simulink model "shifter_system_sim"  (R2018a)
settings: Solver=VariableStepAuto  StartTime=0.0  StopTime=3  RelTol=1e-3
libraries: simulink x2, dspstat3 x1
settings Model: Creator=m_tam  LastModifiedBy=m_tam

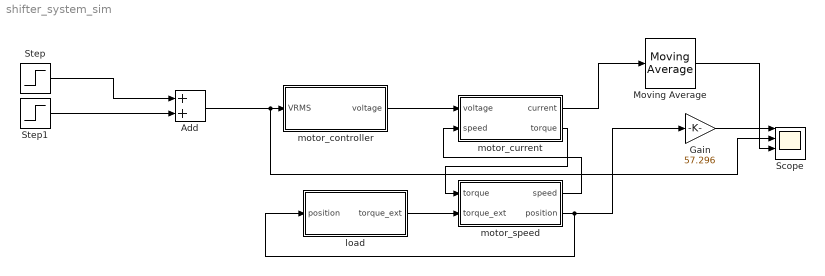
== system shifter_system_sim ==
  Add : Sum
  Gain : Gain  Gain=57.296
  Moving Average : dspstat3/Moving Average  Method=Exponential weighting  ForgettingFactorPort=off  SpecifyWindowLength=on  WindowLength=1000  ForgettingFactor=.999  SimulateUsing=Code generation
  Scope : Scope  NumInputPorts=4
  Step : Step  After=1.125  SampleTime=0
  Step1 : Step  Time=2  After=3  SampleTime=0
  load : Subsystem
  motor_controller : Subsystem
  motor_current : Subsystem
  motor_speed : Subsystem
  wires:
  motor_speed/1(speed) -> motor_current/2(speed)
  motor_speed/2(position) -> load/1(position), Gain/1
  motor_current/2(torque) -> motor_speed/1(torque)
  load/1(torque_ext) -> motor_speed/2(torque_ext)
  motor_controller/1(voltage) -> motor_current/1(voltage)
  Add/1 -> Scope/2, motor_controller/1(VRMS)
  motor_current/1(current) -> Moving Average/1
  Moving Average/1 -> Scope/3
  Gain/1 -> Scope/1
  Step/1 -> Add/1
  Step1/1 -> Add/2

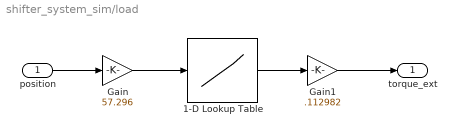
== system shifter_system_sim/load ==
  position : Inport
  1-D Lookup Table : Lookup_n-D  NumberOfTableDimensions=1  BreakpointsForDimension1=[0, 0.01, 57.99, 58]  Table=[20, 6.9, 8.62, 20]  InternalRulePriority=Speed  RndMeth=Simplest  InputSameDT=on
  Gain : Gain  Gain=57.296
  Gain1 : Gain  Gain=.112982
  torque_ext : Outport
  wires:
  position/1 -> Gain/1
  1-D Lookup Table/1 -> Gain1/1
  Gain/1 -> 1-D Lookup Table/1
  Gain1/1 -> torque_ext/1

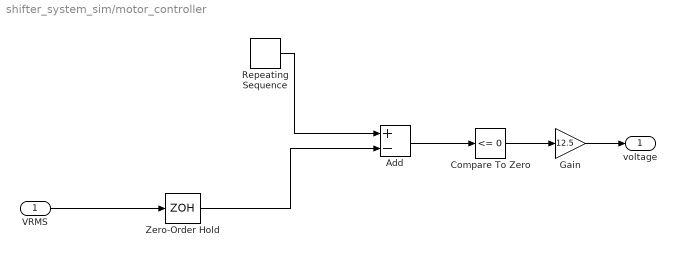
== system shifter_system_sim/motor_controller ==
  VRMS : Inport
  Add : Sum  Inputs=+-
  Compare To Zero : simulink/Logic and Bit Operations/Compare To Zero  relop=<=  OutDataTypeStr=boolean
  Gain : Gain  Gain=12.5
  Repeating Sequence : simulink/Sources/Repeating Sequence  rep_seq_t=[0 .01]  rep_seq_y=[0 5]
  Zero-Order Hold : ZeroOrderHold  SampleTime=.01
  voltage : Outport
  wires:
  VRMS/1 -> Zero-Order Hold/1
  Zero-Order Hold/1 -> Add/2
  Repeating Sequence/1 -> Add/1
  Compare To Zero/1 -> Gain/1
  Add/1 -> Compare To Zero/1
  Gain/1 -> voltage/1

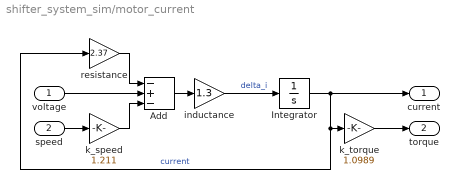
== system shifter_system_sim/motor_current ==
  voltage : Inport
  speed : Inport  Port=2
  Add : Sum  Inputs=-+-
  Integrator : Integrator
  inductance : Gain  Gain=1.3
  k_speed : Gain  Gain=1.211
  k_torque : Gain  Gain=1.0989
  resistance : Gain  Gain=2.37
  current : Outport
  torque : Outport  Port=2
  wires:
  speed/1 -> k_speed/1
  Add/1 -> inductance/1
  inductance/1 -> Integrator/1  "delta_i"
  voltage/1 -> Add/2
  k_speed/1 -> Add/3
  resistance/1 -> Add/1
  Integrator/1 -> resistance/1, k_torque/1, current/1  "current"
  k_torque/1 -> torque/1

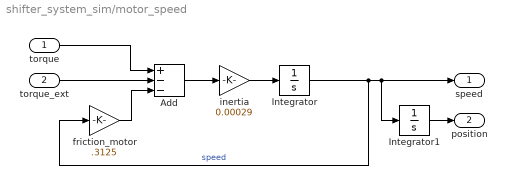
== system shifter_system_sim/motor_speed ==
  torque : Inport
  torque_ext : Inport  Port=2
  Add : Sum  Inputs=+--
  Integrator : Integrator
  Integrator1 : Integrator
  friction_motor : Gain  Gain=.3125
  inertia : Gain  Gain=0.00029
  speed : Outport
  position : Outport  Port=2
  wires:
  torque/1 -> Add/1
  torque_ext/1 -> Add/2
  Add/1 -> inertia/1
  inertia/1 -> Integrator/1
  Integrator/1 -> friction_motor/1, Integrator1/1, speed/1  "speed"
  Integrator1/1 -> position/1
  friction_motor/1 -> Add/3
